simulink model "FF_Kalman_Without_Init"  (R2014a)
settings: Solver=FixedStepDiscrete  SolverMode=SingleTasking  StartTime=1  StopTime=T_end  FixedStep=T  RelTol=1e-3
model workspace: external: MATLAB File (data not in the file)
values from neighbouring files (symbols this model uses):
  A = [exp(-1/tau1)  0 ;      0        exp(-1/tau2)]    [Kal_err.m]
  B = [b1 ; b2 ]    [Kal_err.m]
  base_perf = Out(1)    [Kal_err.m]
  C = [k1 , -k2]    [Kal_err.m]
  M_0 = Q    [Kal_err.m]
  Q = sigma_Sx^2 * [1 0;0 1]    [Kal_err.m]
  R = sigma_Px^2    (= 0.00015876)    [Kal_err.m]
  u_k = In    [Kal_err.m]
  x0hat = [x(6) , x(7)]'    [Kal_err.m]
  x_0 = [x(6) , x(7)]'    [Kal_err.m]
settings Model: Creator=dorothea  LastModifiedBy=Abdullah
settings DataIOCC: ExternalInput=[t, u_k],[t,yout_k]  LoadExternalInput=on  SaveFormat=Structure  ReturnWorkspaceOutputs=on
settings OptimizationCC: BlockReduction=off  BooleanDataType=off  SimCompilerOptimization=off
settings DebuggingCC: SaveWithParameterizedLinksMsg=none  UnderspecifiedInitializationDetection=Classic  SignalResolutionControl=TryResolveAllWithWarning  SolverPrmCheckMsg=none  FrameProcessingCompatibilityMsg=error
settings HardwareCC: TargetUnknown=on
settings RTWCC: RTWCompilerOptimization=off

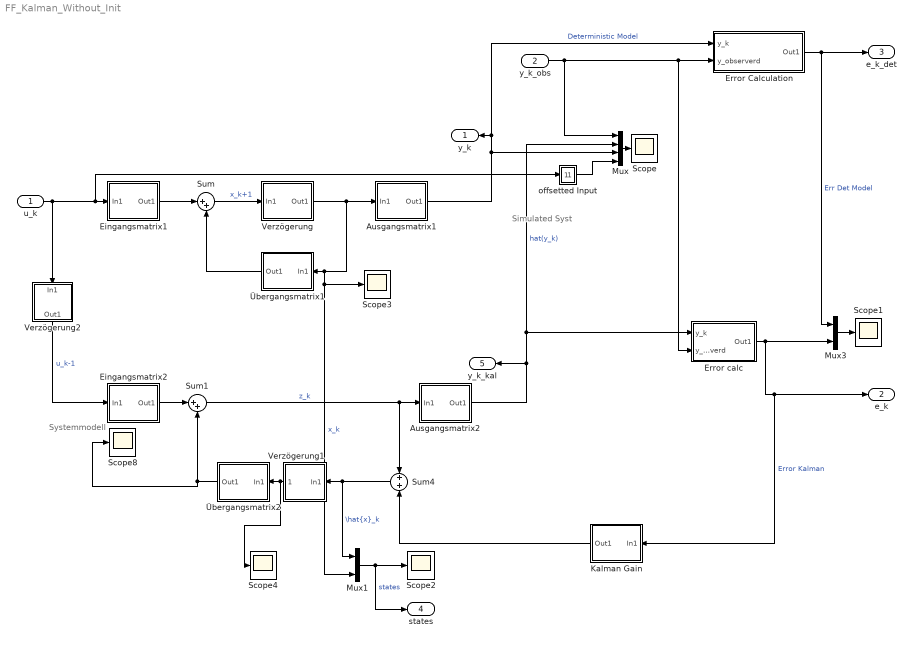
== system FF_Kalman_Without_Init ==
  note: Systemmodell
  note: Simulated Syst
  u_k : Inport
  y_k_obs : Inport  Port=2
  Ausgangsmatrix1 : Subsystem
      mask Display: fprintf('C')
  Ausgangsmatrix2 : Subsystem
      mask Display: fprintf('C')
  Eingangsmatrix1 : Subsystem
      mask Display: fprintf('B')
  Eingangsmatrix2 : Subsystem
      mask Display: fprintf('B')
  Error Calculation : Subsystem
  Error calc : Subsystem
  Kalman Gain : Subsystem
      mask Display: fprintf('K')
  Mux : Mux
      settings: DisplayOption=signals
  Mux1 : Mux  Inputs=2
  Mux3 : Mux  Inputs=2
      settings: DisplayOption=signals
  Scope{,1..4,8} (6 alike) : Scope
      Scope settings: ShowLegends=on  YMin=-1.25  YMax=1.25
      Scope1 settings: ShowLegends=on
      Scope2 settings: ShowLegends=on  SaveName=ScopeData2
      Scope3 settings: SaveName=ScopeData3
      Scope4 settings: ShowLegends=on  SaveName=ScopeData4
      Scope8 settings: ShowLegends=on  SaveName=ScopeData8
  Sum : Sum  Inputs=|++
  Sum1 : Sum  Inputs=|++
  Sum4 : Sum  Inputs=+|+
  Verzögerung : Subsystem
      mask Display: fprintf('T')
  Verzögerung1 : Subsystem
      mask Display: fprintf('T')
  Verzögerung2 : Subsystem
      mask Display: fprintf('T')
  offsetted Input : Subsystem
  Übergangsmatrix1 : Subsystem
      mask Display: fprintf('A')
  Übergangsmatrix2 : Subsystem
      mask Display: fprintf('A')
  y_k : Outport
  e_k : Outport  Port=2
  e_k_det : Outport  Port=3
  states : Outport  Port=4
  y_k_kal : Outport  Port=5
  wires:
  u_k/1 -> offsetted Input/1(In1), Eingangsmatrix1/1(In1), Verzögerung2/1(In1)
  Sum/1 -> Verzögerung/1(In1)  "x_k+1"
  Verzögerung/1(Out1) -> Ausgangsmatrix1/1(In1), Übergangsmatrix1/1(In1), Scope3/1, Mux1/2  "x_k"
  Übergangsmatrix1/1(Out1) -> Sum/2
  Sum1/1 -> Ausgangsmatrix2/1(In1), Sum4/1  "z_k"
  Verzögerung2/1(Out1) -> Eingangsmatrix2/1(In1)  "u_k-1"
  Eingangsmatrix2/1(Out1) -> Sum1/1
  Ausgangsmatrix2/1(Out1) -> y_k_kal/1, Mux/2, Error calc/1(y_k)  "hat(y_k)"
  Verzögerung1/1(Out1) -> Scope4/1, Übergangsmatrix2/1(In1)
  Übergangsmatrix2/1(Out1) -> Sum1/2, Scope8/1
  Sum4/1 -> Verzögerung1/1(In1), Mux1/1  "\\hat{x}_k"
  Kalman Gain/1(Out1) -> Sum4/2
  Mux/1 -> Scope/1
  Mux1/1 -> states/1, Scope2/1  "states"
  Ausgangsmatrix1/1(Out1) -> Error Calculation/1(y_k), y_k/1, Mux/3  "Deterministic Model"
  y_k_obs/1 -> Error Calculation/2(y_observerd), Error calc/2(y_observerd), Mux/1
  offsetted Input/1(Out1) -> Mux/4
  Error Calculation/1(Out1) -> e_k_det/1, Mux3/1  "Err Det Model"
  Mux3/1 -> Scope1/1
  Eingangsmatrix1/1(Out1) -> Sum/1
  Error calc/1(Out1) -> Kalman Gain/1(In1), e_k/1, Mux3/2  "Error Kalman"

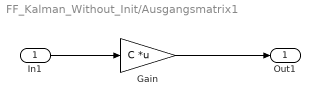
== system FF_Kalman_Without_Init/Ausgangsmatrix1 ==
  In1 : Inport
  Gain : Gain  Gain=C  Multiplication=Matrix(K*u)
  Out1 : Outport
  wires:
  Gain/1 -> Out1/1
  In1/1 -> Gain/1

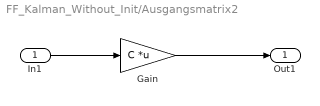
== system FF_Kalman_Without_Init/Ausgangsmatrix2 ==
  In1 : Inport
  Gain : Gain  Gain=C  Multiplication=Matrix(K*u)
  Out1 : Outport
  wires:
  In1/1 -> Gain/1
  Gain/1 -> Out1/1

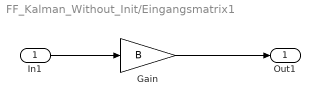
== system FF_Kalman_Without_Init/Eingangsmatrix1 ==
  In1 : Inport
  Gain : Gain  Gain=B
  Out1 : Outport
  wires:
  In1/1 -> Gain/1
  Gain/1 -> Out1/1

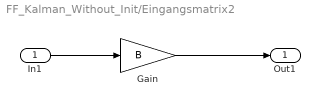
== system FF_Kalman_Without_Init/Eingangsmatrix2 ==
  In1 : Inport
  Gain : Gain  Gain=B
  Out1 : Outport
  wires:
  Gain/1 -> Out1/1
  In1/1 -> Gain/1

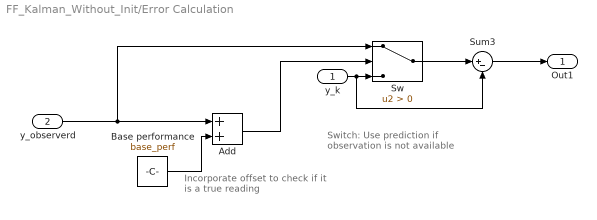
== system FF_Kalman_Without_Init/Error Calculation ==
  note: Incorporate offset to check if it is a true reading
  note: Switch: Use prediction
      | if observation is not available
  y_k : Inport
  y_observerd : Inport  Port=2
  Add : Sum
  Base performance : Constant  Value=base_perf
  Sum3 : Sum  Inputs=|+-
  Sw : Switch  Criteria=u2 > Threshold
  Out1 : Outport
  wires:
  y_observerd/1 -> Sw/1, Add/1
  Base performance/1 -> Add/2
  y_k/1 -> Sum3/2, Sw/3
  Sw/1 -> Sum3/1
  Sum3/1 -> Out1/1
  Add/1 -> Sw/2

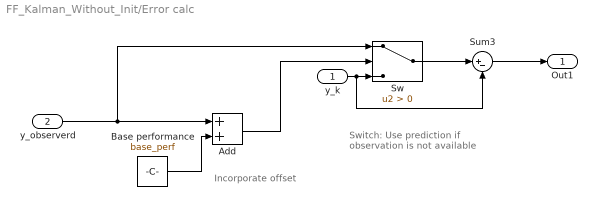
== system FF_Kalman_Without_Init/Error calc ==
  note: Incorporate offset
  note: Switch: Use prediction
      | if observation is not available
  y_k : Inport
  y_observerd : Inport  Port=2
  Add : Sum
  Base performance : Constant  Value=base_perf
  Sum3 : Sum  Inputs=|+-
  Sw : Switch  Criteria=u2 > Threshold
  Out1 : Outport
  wires:
  y_observerd/1 -> Sw/1, Add/1
  Base performance/1 -> Add/2
  y_k/1 -> Sum3/2, Sw/3
  Sw/1 -> Sum3/1
  Sum3/1 -> Out1/1
  Add/1 -> Sw/2

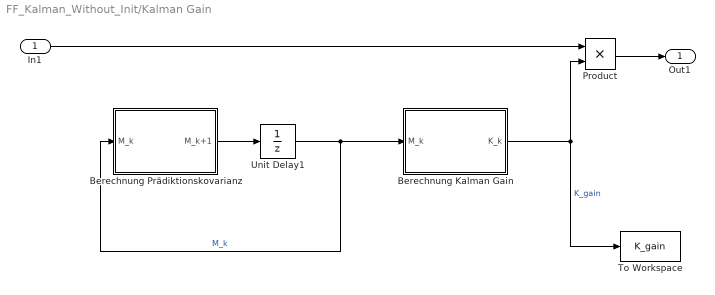
== system FF_Kalman_Without_Init/Kalman Gain ==
  In1 : Inport
  Berechnung Prädiktionskovarianz : Subsystem
  Berechnung Kalman Gain : Subsystem
  Product : Product  RndMeth=Zero
  To Workspace : ToWorkspace  VariableName=K_gain  SaveFormat=Structure  SampleTime=-1
  Unit Delay1 : UnitDelay  InitialCondition=M_0  SampleTime=-1
  Out1 : Outport
  wires:
  In1/1 -> Product/1
  Product/1 -> Out1/1
  Unit Delay1/1 -> Berechnung Kalman Gain/1(M_k), Berechnung Prädiktionskovarianz/1(M_k)  "M_k"
  Berechnung Prädiktionskovarianz/1(M_k+1) -> Unit Delay1/1
  Berechnung Kalman Gain/1(K_k) -> To Workspace/1, Product/2  "K_gain"

== system FF_Kalman_Without_Init/Verzögerung ==
  In1 : Inport
  Unit Delay : UnitDelay  InitialCondition=x_0  SampleTime=-1
  Out1 : Outport
  wires:
  In1/1 -> Unit Delay/1
  Unit Delay/1 -> Out1/1

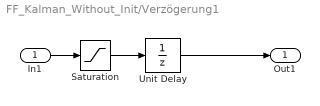
== system FF_Kalman_Without_Init/Verzögerung1 ==
  In1 : Inport
  Saturation : Saturate  UpperLimit=20000  LowerLimit=0  LinearizeAsGain=off  OutMin=0  OutMax=20000
  Unit Delay : UnitDelay  InitialCondition=x0hat  SampleTime=-1
  Out1 : Outport
  wires:
  In1/1 -> Saturation/1
  Unit Delay/1 -> Out1/1
  Saturation/1 -> Unit Delay/1

== system FF_Kalman_Without_Init/Verzögerung2 ==
  In1 : Inport
  Unit Delay : UnitDelay  SampleTime=-1
  Out1 : Outport
  wires:
  In1/1 -> Unit Delay/1
  Unit Delay/1 -> Out1/1

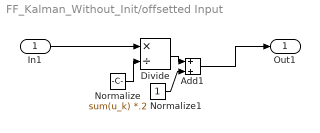
== system FF_Kalman_Without_Init/offsetted Input ==
  In1 : Inport
  Add1 : Sum
  Divide : Product  Inputs=*/
  Normalize : Constant  Value=sum(u_k) *.2
  Normalize1 : Constant
  Out1 : Outport
  wires:
  Normalize/1 -> Divide/2
  Divide/1 -> Add1/1
  Normalize1/1 -> Add1/2
  In1/1 -> Divide/1
  Add1/1 -> Out1/1

== system FF_Kalman_Without_Init/Übergangsmatrix1 ==
  In1 : Inport
  Gain : Gain  Gain=A  Multiplication=Matrix(K*u)
  Out1 : Outport
  wires:
  Gain/1 -> Out1/1
  In1/1 -> Gain/1

== system FF_Kalman_Without_Init/Übergangsmatrix2 ==
  In1 : Inport
  Gain : Gain  Gain=A  Multiplication=Matrix(K*u)
  Out1 : Outport
  wires:
  In1/1 -> Gain/1
  Gain/1 -> Out1/1

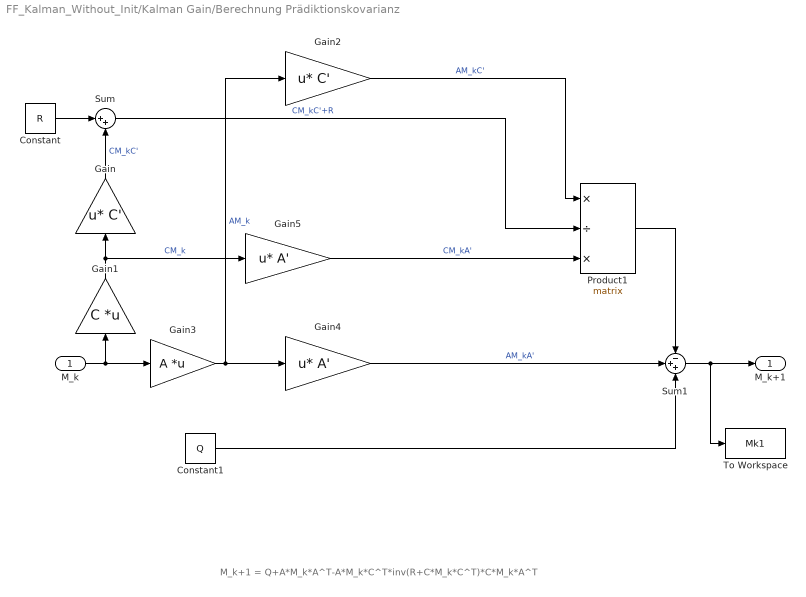
== system FF_Kalman_Without_Init/Kalman Gain/Berechnung Prädiktionskovarianz ==
  note: M_k+1 = Q+A*M_k*A^T-A*M_k*C^T*inv(R+C*M_k*C^T)*C*M_k*A^T
  M_k : Inport
  Constant : Constant  Value=R
  Constant1 : Constant  Value=Q  VectorParams1D=off
  Gain : Gain  Gain=C'  Multiplication=Matrix(u*K)
  Gain1 : Gain  Gain=C  Multiplication=Matrix(K*u)
  Gain2 : Gain  Gain=C'  Multiplication=Matrix(u*K)
  Gain3 : Gain  Gain=A  Multiplication=Matrix(K*u)
  Gain4 : Gain  Gain=A'  Multiplication=Matrix(u*K)
  Gain5 : Gain  Gain=A'  Multiplication=Matrix(u*K)
  Product1 : Product  Inputs=*/*  Multiplication=Matrix(*)  RndMeth=Zero
  Sum : Sum  Inputs=|++
  Sum1 : Sum  Inputs=-++
  To Workspace : ToWorkspace  VariableName=Mk1  SaveFormat=Structure  SampleTime=-1
  M_k+1 : Outport
  wires:
  Gain/1 -> Sum/2  "CM_kC'"
  Gain1/1 -> Gain/1, Gain5/1  "CM_k"
  Constant/1 -> Sum/1
  M_k/1 -> Gain3/1, Gain1/1
  Gain3/1 -> Gain4/1, Gain2/1  "AM_k"
  Gain2/1 -> Product1/1  "AM_kC'"
  Sum/1 -> Product1/2  "CM_kC'+R"
  Gain5/1 -> Product1/3  "CM_kA'"
  Product1/1 -> Sum1/1
  Gain4/1 -> Sum1/2  "AM_kA'"
  Constant1/1 -> Sum1/3
  Sum1/1 -> M_k+1/1, To Workspace/1

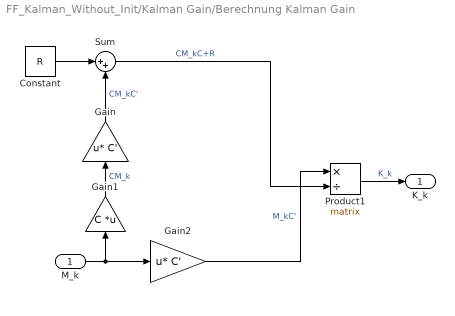
== system FF_Kalman_Without_Init/Kalman Gain/Berechnung Kalman Gain ==
  M_k : Inport
  Constant : Constant  Value=R
  Gain : Gain  Gain=C'  Multiplication=Matrix(u*K)
  Gain1 : Gain  Gain=C  Multiplication=Matrix(K*u)
  Gain2 : Gain  Gain=C'  Multiplication=Matrix(u*K)
  Product1 : Product  Inputs=*/  Multiplication=Matrix(*)  RndMeth=Zero
  Sum : Sum  Inputs=|++
  K_k : Outport
  wires:
  M_k/1 -> Gain2/1, Gain1/1
  Constant/1 -> Sum/1
  Gain1/1 -> Gain/1  "CM_k"
  Gain/1 -> Sum/2  "CM_kC'"
  Gain2/1 -> Product1/1  "M_kC'"
  Sum/1 -> Product1/2  "CM_kC+R"
  Product1/1 -> K_k/1  "K_k"
